simulink model "Fig210"  (R2014b)
settings: Solver=ode3  StartTime=0.0  StopTime=10.001  FixedStep=2e-5  RelTol=1e-5
libraries: commchan3 x1, commsink2 x1, dsparch4 x1, commrandsrc2 x1, dspsigops x1
settings Model: Creator=Dennis Silage  LastModifiedBy=Silage
settings DataIOCC: SignalLoggingSaveFormat=ModelDataLogs
settings OptimizationCC: ExpressionDepthLimit=2147483647  InitFltsAndDblsToZero=on
settings DebuggingCC: UnderspecifiedInitializationDetection=Classic  MergeDetectMultiDrivingBlocksExec=none  SolverPrmCheckMsg=none  FcnCallInpInsideContextMsg=UseLocalSettings  StateNameClashWarn=warning
settings GRTTargetCC: CombineOutputUpdateFcns=off  GRTInterface=on

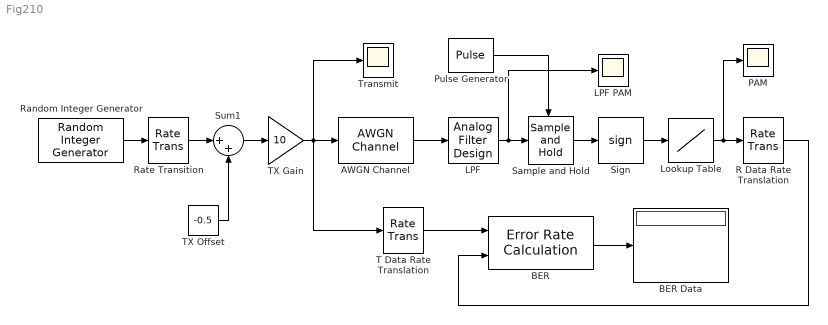
== system Fig210 ==
  AWGN Channel : commchan3/AWGN Channel  InputProcessing=Inherited (this choice will be removed - see release notes)  seed=randseed  noiseMode=Variance from mask  EbNodB=10  EsNodB=10  SNRdB=10  bitsPerSym=1  Ps=1  Tsym=1  variance=0
  BER : commsink2/Error Rate Calculation  N=2  st_delay=0  cp_mode=Entire frame  subframe=[]  PMode=Port  WsName=ErrorVec  RsMode2=off  stop=off  numErr=100  maxBits=1e6
  BER Data : Display
  LPF : dsparch4/Analog Filter Design  method=Chebyshev I  filttype=Lowpass  N=9  Wlo=2*pi*1200  Whi=80  Rp=0.1  Rs=40
  LPF PAM : Scope
      settings: TimeRange=0.05  YMin=-8  YMax=8  SaveName=ScopeData2
  Lookup Table : Lookup_n-D  NumberOfTableDimensions=1  BreakpointsForDimension1=[-1,0,1]  BreakpointsForDimension3=[5, 7]  Table=[-5,5,5]  InternalRulePriority=Speed  RndMeth=Simplest  InputSameDT=on
  PAM : Scope
      settings: TimeRange=0.05  YMin=-8  YMax=8
  Pulse Generator : DiscretePulseGenerator  PulseType=Time based  Period=1e-3  PulseWidth=10  PhaseDelay=5e-4
  R Data Rate Translation : RateTransition  OutPortSampleTime=1e-3
  Random Integer Generator : commrandsrc2/Random Integer Generator  mul=2  seed=randseed  Ts=1e-3  frameBased=off  sampPerFrame=50  orient=on  outDataType=double
  Rate Transition : RateTransition  OutPortSampleTime=2e-5
  Sample and Hold : dspsigops/Sample and Hold  trig=Rising edge  initCond=0  latchinput=off
  Sign : Signum
  Sum1 : Sum  Inputs=|++
  T Data Rate Translation : RateTransition  OutPortSampleTime=1e-3
  TX Gain : Gain  Gain=10
  TX Offset : Constant  Value=-0.5
  Transmit : Scope
      settings: TimeRange=0.05  YMin=-8  YMax=8
  wires:
  Pulse Generator/1 -> Sample and Hold/Trigger
  TX Gain/1 -> T Data Rate Translation/1, Transmit/1, AWGN Channel/1
  Sign/1 -> Lookup Table/1
  Random Integer Generator/1 -> Rate Transition/1
  Rate Transition/1 -> Sum1/1
  Sum1/1 -> TX Gain/1
  TX Offset/1 -> Sum1/2
  Sample and Hold/1 -> Sign/1
  R Data Rate Translation/1 -> BER/2
  BER/1 -> BER Data/1
  Lookup Table/1 -> R Data Rate Translation/1, PAM/1
  T Data Rate Translation/1 -> BER/1
  AWGN Channel/1 -> LPF/1
  LPF/1 -> Sample and Hold/1, LPF PAM/1
